simulink model "gm_VSD_and_Park_transformation_6Phase"  (R2022a)
settings: Solver=FixedStepDiscrete  StartTime=0.0  StopTime=0.2  RelTol=1e-3
libraries: hdlmdlgenlib x2
(part 2 of 2)

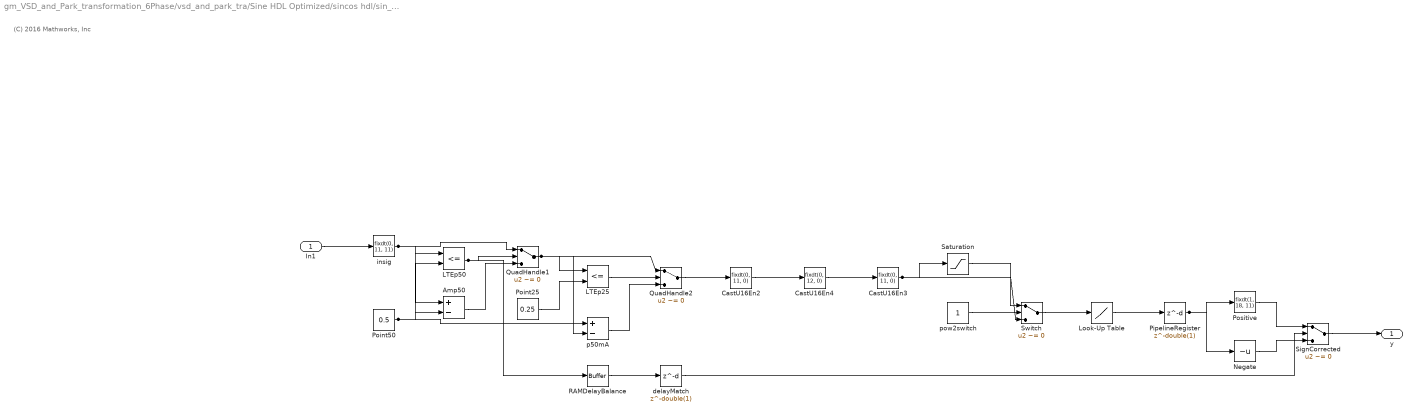
== system gm_VSD_and_Park_transformation_6Phase/vsd_and_park_tra/Sine HDL Optimized/sincos hdl/sin_hdl ==
  note: (C) 2016 Mathworks, Inc
  In1 : Inport  OutDataTypeStr=fixdt(1, 48, 45)  SampleTime=1e-08
  Amp50 : Sum  Inputs=+-  AccumDataTypeStr=fixdt(1, 19, 18)  OutDataTypeStr=fixdt(1, 19, 18)  SampleTime=1e-08
  CastU16En2 : DataTypeConversion  OutDataTypeStr=fixdt(0, 11, 0)  ConvertRealWorld=Stored Integer (SI)  SampleTime=1e-08  SaturateOnIntegerOverflow=off  RndMeth=Floor
  CastU16En3 : DataTypeConversion  OutDataTypeStr=fixdt(0, 11, 0)  ConvertRealWorld=Stored Integer (SI)  SampleTime=1e-08  RndMeth=Floor
  CastU16En4 : DataTypeConversion  OutDataTypeStr=fixdt(0, 12, 0)  SampleTime=1e-08  SaturateOnIntegerOverflow=off  RndMeth=Floor
  LTEp25 : RelationalOperator  Operator=<=  OutDataTypeStr=boolean  SampleTime=1e-08  InputSameDT=off
  LTEp50 : RelationalOperator  Operator=<=  OutDataTypeStr=boolean  SampleTime=1e-08  InputSameDT=off
  Look-Up Table : Lookup_n-D  NumberOfTableDimensions=1  BreakpointsForDimension1="fi(\"numerictype\",numerictype(0,11,0),\"fimath\",fimath(\"RoundingMethod\", \"Floor\",\"OverflowAction\", \"Wrap\",\"ProductMode\",\"FullPrecision\",\"SumMode\",\"FullPrecision\"),\"Value\",\"[0 1 2 3 4 5 6 7 8 9 10 11 12 13 14 15 16 17 18 19 20 21 22 23 24 25 26 27 28 29 30 31 32 33 34 35 36 37 38 39 40 41 42 43 44 45 46 47 48 49 50 51 52 53 54 55 56 57 58 59 60 61 62 63 64 65 66 67 68 69 70 71 72 73 74 75 76 77 78 79 80 81 82 83 84 85 86 87 88 89 90 91 92 93 94 95 96 97 98 99 100 101 102 103 104 105 106 107 108 109 110 111 112 113 114 115 116 117 118 119 120 121 122 123 124 125 126 127 128 129 130 131 132 133 134 135 136 137 138 139 140 141 142 143 144 145 146 147 148 149 150 151 152 153 154 155 156 157 158 159 160 161 162 163 164 165 166 167 168 169 170 171 172 173 174 175 176 177 178 179 180 181 182 183 184 185 186 187 188 189 190 191 192 193 194 195 196 197 198 199 200 201 202 203 204 205 206 207 208 209 210 211 212 213 214 215 216 217 218 219 220 221 222 223 224 225 226 227 228 229 230 231 232 233 234 235 236 237 238 239 240 241 242 243 244 245 246 247 248 249 250 251 252 253 254 255 256 257 258 259 260 261 262 263 264 265 266 267 268 269 270 271 272 273 274 275 276 277 278 279 280 281 282 283 284 285 286 287 288 289 290 291 292 293 294 295 296 297 298 299 300 301 302 303 304 305 306 307 308 309 310 311 312 313 314 315 316 317 318 319 320 321 322 323 324 325 326 327 328 329 330 331 332 333 334 335 336 337 338 339 340 341 342 343 344 345 346 347 348 349 350 351 352 353 354 355 356 357 358 359 360 361 362 363 364 365 366 367 368 369 370 371 372 373 374 375 376 377 378 379 380 381 382 383 384 385 386 387 388 389 390 391 392 393 394 395 396 397 398 399 400 401 402 403 404 405 406 407 408 409 410 411 412 413 414 415 416 417 418 419 420 421 422 423 424 425 426 427 428 429 430 431 432 433 434 435 436 437 438 439 440 441 442 443 444 445 446 447 448 449 450 451 452 453 454 455 456 457 458 459 460 461 462 463 464 465 466 467 468 469 470 471 472 473 474 475 476 477 478 479 480 481 482 483 484 485 486 487 488 489 490 491 492 493 494 495 496 497 498 499 500 501 502 503 504 505 506 507 508 509 510 511]\")"  Table="reshape(fi(\"numerictype\",numerictype(1,18,11),\"fimath\",fimath(\"RoundingMethod\", \"Floor\",\"OverflowAction\", \"Wrap\",\"ProductMode\",\"FullPrecision\",\"SumMode\",\"FullPrecision\"),\"Value\",\"[0;0.0029296875;0.00634765625;0.00927734375;0.01220703125;0.01513671875;0.0185546875;0.021484375;0.0244140625;0.02783203125;0.03076171875;0.03369140625;0.037109375;0.0400390625;0.04296875;0.0458984375;0.04931640625;0.05224609375;0.05517578125;0.05859375;0.0615234375;0.064453125;0.0673828125;0.07080078125;0.07373046875;0.07666015625;0.080078125;0.0830078125;0.0859375;0.0888671875;0.09228515625;0.09521484375;0.09814453125;0.10107421875;0.1044921875;0.107421875;0.1103515625;0.11328125;0.11669921875;0.11962890625;0.12255859375;0.12548828125;0.12890625;0.1318359375;0.134765625;0.1376953125;0.14111328125;0.14404296875;0.14697265625;0.14990234375;0.1533203125;0.15625;0.1591796875;0.162109375;0.1650390625;0.16845703125;0.17138671875;0.17431640625;0.17724609375;0.18017578125;0.18359375;0.1865234375;0.189453125;0.1923828125;0.1953125;0.1982421875;0.20166015625;0.20458984375;0.20751953125;0.21044921875;0.21337890625;0.21630859375;0.2197265625;0.22265625;0.2255859375;0.228515625;0.2314453125;0.234375;0.2373046875;0.240234375;0.24365234375;0.24658203125;0.24951171875;0.25244140625;0.25537109375;0.25830078125;0.26123046875;0.26416015625;0.26708984375;0.27001953125;0.27294921875;0.27587890625;0.27880859375;0.2822265625;0.28515625;0.2880859375;0.291015625;0.2939453125;0.296875;0.2998046875;0.302734375;0.3056640625;0.30859375;0.3115234375;0.314453125;0.3173828125;0.3203125;0.3232421875;0.32568359375;0.32861328125;0.33154296875;0.33447265625;0.33740234375;0.34033203125;0.34326171875;0.34619140625;0.34912109375;0.35205078125;0.35498046875;0.35791015625;0.3603515625;0.36328125;0.3662109375;0.369140625;0.3720703125;0.375;0.3779296875;0.38037109375;0.38330078125;0.38623046875;0.38916015625;0.39208984375;0.39453125;0.3974609375;0.400390625;0.4033203125;0.40576171875;0.40869140625;0.41162109375;0.41455078125;0.4169921875;0.419921875;0.4228515625;0.42578125;0.42822265625;0.43115234375;0.43408203125;0.4365234375;0.439453125;0.4423828125;0.44482421875;0.44775390625;0.4501953125;0.453125;0.4560546875;0.45849609375;0.46142578125;0.4638671875;0.466796875;0.4697265625;0.47216796875;0.47509765625;0.4775390625;0.48046875;0.48291015625;0.48583984375;0.48828125;0.4912109375;0.49365234375;0.49658203125;0.4990234375;0.501953125;0.50439453125;0.50732421875;0.509765625;0.51220703125;0.51513671875;0.517578125;0.5205078125;0.52294921875;0.525390625;0.5283203125;0.53076171875;0.533203125;0.5361328125;0.53857421875;0.541015625;0.54345703125;0.54638671875;0.548828125;0.55126953125;0.55419921875;0.556640625;0.55908203125;0.5615234375;0.56396484375;0.56689453125;0.5693359375;0.57177734375;0.57421875;0.57666015625;0.5791015625;0.58203125;0.58447265625;0.5869140625;0.58935546875;0.591796875;0.59423828125;0.5966796875;0.59912109375;0.6015625;0.60400390625;0.6064453125;0.60888671875;0.611328125;0.61376953125;0.6162109375;0.61865234375;0.62109375;0.62353515625;0.6259765625;0.62841796875;0.630859375;0.6328125;0.63525390625;0.6376953125;0.64013671875;0.642578125;0.64501953125;0.6474609375;0.6494140625;0.65185546875;0.654296875;0.65673828125;0.65869140625;0.6611328125;0.66357421875;0.666015625;0.66796875;0.67041015625;0.6728515625;0.6748046875;0.67724609375;0.67919921875;0.681640625;0.68408203125;0.68603515625;0.6884765625;0.6904296875;0.69287109375;0.69482421875;0.697265625;0.69921875;0.70166015625;0.70361328125;0.7060546875;0.7080078125;0.71044921875;0.71240234375;0.71484375;0.716796875;0.71875;0.72119140625;0.72314453125;0.72509765625;0.7275390625;0.7294921875;0.7314453125;0.73388671875;0.73583984375;0.73779296875;0.73974609375;0.7421875;0.744140625;0.74609375;0.748046875;0.75;0.75244140625;0.75439453125;0.75634765625;0.75830078125;0.76025390625;0.76220703125;0.76416015625;0.76611328125;0.76806640625;0.77001953125;0.77197265625;0.77392578125;0.77587890625;0.77783203125;0.77978515625;0.78173828125;0.78369140625;0.78564453125;0.78759765625;0.78955078125;0.79150390625;0.79296875;0.794921875;0.796875;0.798828125;0.80078125;0.80224609375;0.80419921875;0.80615234375;0.80810546875 ...(+2575 chars)]\"), [1  512])"  InterpMethod=Flat  ExtrapMethod=Clip  DiagnosticForOutOfRangeInput=Error  SampleTime=1e-08  OutDataTypeStr=fixdt(1, 18, 11)
  Negate : UnaryMinus  SampleTime=1e-08
  PipelineRegister : Delay  DelayLength=double(1)  InitialCondition=0  SampleTime=1e-08
  Point25 : Constant  Value=0.25  OutDataTypeStr=fixdt(0, 18, 18)  SampleTime=1e-08
  Point50 : Constant  Value=0.5  OutDataTypeStr=fixdt(0, 18, 18)  SampleTime=1e-08
  Positive : DataTypeConversion  OutDataTypeStr=fixdt(1, 18, 11)  SampleTime=1e-08  SaturateOnIntegerOverflow=off  RndMeth=Floor
  QuadHandle1 : Switch  Criteria=u2 ~= 0  Threshold=double(0)  OutDataTypeStr=fixdt(1, 19, 18)  SampleTime=1e-08  SaturateOnIntegerOverflow=off  InputSameDT=off
  QuadHandle2 : Switch  Criteria=u2 ~= 0  Threshold=double(0)  OutDataTypeStr=fixdt(0, 11, 11)  SampleTime=1e-08  SaturateOnIntegerOverflow=off  InputSameDT=off
  RAMDelayBalance : hdlmdlgenlib/Buffer
      settings: SourceProductBaseCode=SL
  Saturation : Saturate  UpperLimit="fi(0,0,11,0,\"hex\",\"1ff\")"  LowerLimit="fi(0,0,11,0,\"hex\",\"000\")"  SampleTime=1e-08  OutDataTypeStr=fixdt(0, 11, 0)
  SignCorrected : Switch  Criteria=u2 ~= 0  Threshold=double(0)  OutDataTypeStr=fixdt(1, 18, 11)  SampleTime=1e-08  SaturateOnIntegerOverflow=off  InputSameDT=off
  Switch : Switch  Criteria=u2 ~= 0  Threshold=double(0)  OutDataTypeStr=fixdt(0, 11, 0)  SampleTime=1e-08  SaturateOnIntegerOverflow=off  InputSameDT=off
  delayMatch : Delay  DelayLength=double(1)  InitialCondition=0  SampleTime=1e-08
  insig : DataTypeConversion  OutDataTypeStr=fixdt(0, 11, 11)  SampleTime=1e-08  SaturateOnIntegerOverflow=off  RndMeth=Floor
  p50mA : Sum  Inputs=+-  AccumDataTypeStr=fixdt(1, 20, 18)  OutDataTypeStr=fixdt(1, 20, 18)  SampleTime=1e-08
  pow2switch : Constant  OutDataTypeStr=boolean  SampleTime=1e-08
  y : Outport  SampleTime=1e-08
  wires:
  Amp50/1 -> QuadHandle1/3
  CastU16En2/1 -> CastU16En4/1
  CastU16En3/1 -> Switch/3, Saturation/1
  CastU16En4/1 -> CastU16En3/1
  LTEp25/1 -> QuadHandle2/2
  LTEp50/1 -> QuadHandle1/2, RAMDelayBalance/1
  PipelineRegister/1 -> Positive/1, Negate/1
  Negate/1 -> SignCorrected/3
  Point25/1 -> LTEp25/2
  Point50/1 -> p50mA/1, LTEp50/2, Amp50/2
  Positive/1 -> SignCorrected/1
  QuadHandle1/1 -> p50mA/2, QuadHandle2/1, LTEp25/1
  QuadHandle2/1 -> CastU16En2/1
  delayMatch/1 -> SignCorrected/2
  Saturation/1 -> Switch/1
  SignCorrected/1 -> y/1
  Switch/1 -> Look-Up Table/1
  insig/1 -> QuadHandle1/1, LTEp50/1, Amp50/1
  p50mA/1 -> QuadHandle2/3
  pow2switch/1 -> Switch/2
  In1/1 -> insig/1
  RAMDelayBalance/1 -> delayMatch/1
  Look-Up Table/1 -> PipelineRegister/1

== matlab function gm_VSD_and_Park_transformation_6Phase/vsd_and_park_tra/MATLAB Function1/MATLAB Function1 ==
  settings: fimath=fimath('RoundingMethod', 'Floor','OverflowAction', 'Wrap','ProductMode', 'FullPrecision', 'SumMode', 'FullPrecision')
  data: u input; y output
function y = fcn(u)

    y = u*(1/(2*pi));

end

== matlab function gm_VSD_and_Park_transformation_6Phase/vsd_and_park_tra/MATLAB Function/MATLAB Function ==
  settings: fimath=fimath('RoundingMethod', 'Floor','OverflowAction', 'Wrap','ProductMode', 'FullPrecision', 'SumMode', 'FullPrecision')
  data: i_a1 input; i_alpha output; i_b1 input; i_c1 input; i_a2 input; i_b2 input; i_c2 input; sin_theta_el input; i_beta output; i_x output; i_y output; i_0_plus output; i_0_minus output; i_d output; i_q output; cos_theta_el input
function [i_alpha,i_beta,i_x,i_y,i_0_plus,i_0_minus,i_d,i_q] = VSD_and_Park_transformation(i_a1,i_b1,i_c1,i_a2,i_b2,i_c2,sin_theta_el,cos_theta_el)

    % VSD-Transformation
    A = [0 0 0 0 0 0]';

    A =  0.3333*[1    -0.5        -0.5        0.8660   -0.8660  0 ;
                0    0.8660   -0.8660  0.5         0.5         -1;
                1    -0.5        -0.5        -0.8660  0.8660   0 ;
                0    -0.8660  0.8660   0.5         0.5         -1;
                1    1           1           0           0           0 ;
                0    0           0           1           1           1] * [i_a1 i_b1 i_c1 i_a2 i_b2 i_c2]';

    i_alpha = A(1);
    i_beta = A(2);
    i_x = A(3);
    i_y = A(4);
    i_0_plus = A(5);
    i_0_minus = A(6);

    % Park-Transformation
%    B = [0 0]';

%     B = [cos(theta_el)       sin(theta_el);
%         -sin(theta_el)       cos(theta_el)] * [i_alpha i_beta]';

 %   i_d = B(1);
 %   i_q = B(2);



i_d = cos_theta_el*i_alpha+sin_theta_el*i_beta;
i_q = -sin_theta_el*i_alpha+cos_theta_el*i_beta;


end

== matlab function gm_VSD_and_Park_transformation_6Phase/MATLAB Function2 ==
  data: theta_el input; theta_el_with_offset_scaled output; theta_el_offset input
function theta_el_with_offset_scaled = fcn(theta_el, theta_el_offset)

theta_el_with_offset = theta_el-theta_el_offset;


if theta_el_with_offset>=(2*pi)
    theta_el_with_offset_scaled = theta_el_with_offset-2*pi;
else
    theta_el_with_offset_scaled = theta_el_with_offset+0;
end

if theta_el_with_offset<(2*pi)
    theta_el_with_offset_scaled = theta_el_with_offset+2*pi;
end

end
